simulink model "ownStateSpaceModel"  (R2015a)
settings: Solver=ode4  StartTime=0.0  StopTime=100  RelTol=1e-3
values from neighbouring files (symbols this model uses):
  A = M^(-1) * A_prim    [A_B_determinant.m]    (also in A_B_determinant_new.m; A_B_lateral.m = simplify(M^(-1) * A_prim); A_B_lateral_creation.m = simplify(A); RungeKutta2.m = A2)
  B = simplify(M^(-1) * B_prim)    [A_B_lateral.m]    (also in A_B_lateral_creation.m = simplify(B); RungeKutta2.m = B2; check.m = zeros(6))
  C = eye(5)    [AircraftStrategy.m]    (also in MissileStrategy.m = [eye(3), zeros(3); zeros(3,6)])
  x0 = obj.missileState'    [MissileStrategy.m]
undefined symbols (not defined in the file or in its folder): D
settings Model: Creator=adamfelis  LastModifiedBy=Qba

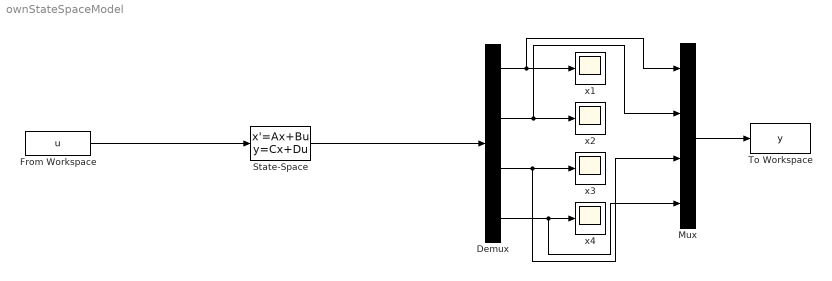
== system ownStateSpaceModel ==
  Demux : Demux
  From Workspace : FromWorkspace  VariableName=u  SampleTime=0
  Mux : Mux
  State-Space : StateSpace  A=A  B=B  C=C  D=D  X0=x0
  To Workspace : ToWorkspace  VariableName=y  SaveFormat=Timeseries  SampleTime=-1
  x{1..4} (4 alike) : Scope
      x3 settings: SaveName=ScopeData2
      x4 settings: SaveName=ScopeData4
  wires:
  State-Space/1 -> Demux/1
  Demux/4 -> Mux/4, x4/1
  Demux/2 -> Mux/2, x2/1
  Demux/1 -> Mux/1, x1/1
  Demux/3 -> Mux/3, x3/1
  Mux/1 -> To Workspace/1
  From Workspace/1 -> State-Space/1
